simulink model "Final_v000"  (R2019b)
settings: Solver=ode4  StartTime=0.0  StopTime=10000  FixedStep=1  RelTol=1e-3
libraries: simulink x7
(part 2 of 2)

== system Final_v000/ポンプ/実H/ベルヌーイの定理/速度ヘッド ==
  v : Inport
  Constant : Constant  Value=2
  Data Store Read1 : DataStoreRead  DataStoreName=g
  Divide : Product  Inputs=*/
  Product : Product
  Square : Math  Operator=square  SignedPower=off  SaturateOnIntegerOverflow=on
  Subtract2 : Sum  Inputs=+-
  Unit Delay : UnitDelay  SampleTime=-1  HasFrameUpgradeWarning=on
  速度ヘッド : Outport
  wires:
  Constant/1 -> Product/1
  v/1 -> Square/1
  Product/1 -> Divide/2
  Unit Delay/1 -> Subtract2/2
  Square/1 -> Unit Delay/1, Subtract2/1
  Data Store Read1/1 -> Product/2
  Divide/1 -> 速度ヘッド/1
  Subtract2/1 -> Divide/1

== system Final_v000/ラジエーター/Q=hAdT/h計算/Nu更新 ==
  note: Nu=3.66 (Re<2000)
      | Nu=0.023・(Re^0.8)・(Pr^0.3) (Re>=2000)
  流量Q : Inport
  Constant : Constant  Value=3.66
  Constant1 : Constant  Value=0.023
  Constant2 : Constant  Value=0.8
  Constant3 : Constant  Value=0.3
  Power : Math  Operator=pow  SignedPower=off  SaturateOnIntegerOverflow=on
  Power1 : Math  Operator=pow  SignedPower=off  SaturateOnIntegerOverflow=on
  Product : Product  Inputs=3
  Pr更新 : Subsystem
  Re更新 : Subsystem
  Switch : Switch  Threshold=2000
  Nu : Outport
  wires:
  Constant/1 -> Switch/3
  Switch/1 -> Nu/1
  Re更新/1(Re) -> Switch/2, Power/1
  Constant2/1 -> Power/2
  Pr更新/1(Pr) -> Power1/1
  Constant3/1 -> Power1/2
  Constant1/1 -> Product/1
  Power/1 -> Product/2
  Power1/1 -> Product/3
  Product/1 -> Switch/1
  流量Q/1 -> Re更新/1(流量Q)

== system Final_v000/エンジン/Q=hAdT/h計算 /Nu更新/Pr更新 ==
  note: Pr=μ・Cp/k
  Data Store Read : DataStoreRead  DataStoreName=Cp
  Data Store Read2 : DataStoreRead  DataStoreName=viscosity
  Data Store Read3 : DataStoreRead  DataStoreName=k
  Divide : Product  Inputs=*/
  Product : Product
  Pr : Outport
  wires:
  Data Store Read2/1 -> Product/2  "μ"
  Data Store Read/1 -> Product/1  "Cp"
  Product/1 -> Divide/1
  Data Store Read3/1 -> Divide/2  "k"
  Divide/1 -> Pr/1  "Pr"

== system Final_v000/エンジン/Q=hAdT/h計算 /Nu更新/Re更新 ==
  note: Re=4ρQ/ΠμD
  流量Q : Inport
  Constant : Constant  Value=4
  Constant1 : Constant  Value=pi
  Data Store Read : DataStoreRead  DataStoreName=density
  Data Store Read2 : DataStoreRead  DataStoreName=viscosity
  Data Store Read3 : DataStoreRead  DataStoreName=D
  Divide : Product  Inputs=*/
  Product : Product  Inputs=3
  Product1 : Product  Inputs=3
  Re : Outport
  wires:
  Constant/1 -> Product/1
  Data Store Read/1 -> Product/2  "ρ"
  流量Q/1 -> Product/3  "Q"
  Product/1 -> Divide/1
  Data Store Read2/1 -> Product1/2  "μ"
  Constant1/1 -> Product1/1
  Data Store Read3/1 -> Product1/3  "D"
  Product1/1 -> Divide/2
  Divide/1 -> Re/1  "Re"

== system Final_v000/ラジエーター/Q=hAdT/h計算/Nu更新/Pr更新 ==
  note: Pr=μ・Cp/k
  Data Store Read : DataStoreRead  DataStoreName=Cp
  Data Store Read2 : DataStoreRead  DataStoreName=viscosity
  Data Store Read3 : DataStoreRead  DataStoreName=k
  Divide : Product  Inputs=*/
  Product : Product
  Pr : Outport
  wires:
  Data Store Read2/1 -> Product/2
  Data Store Read/1 -> Product/1
  Product/1 -> Divide/1
  Data Store Read3/1 -> Divide/2
  Divide/1 -> Pr/1

== system Final_v000/ラジエーター/Q=hAdT/h計算/Nu更新/Re更新 ==
  note: Re=4ρQ/ΠμD
  流量Q : Inport
  Constant : Constant  Value=4
  Constant1 : Constant  Value=pi
  Data Store Read : DataStoreRead  DataStoreName=density
  Data Store Read2 : DataStoreRead  DataStoreName=viscosity
  Data Store Read3 : DataStoreRead  DataStoreName=D
  Divide : Product  Inputs=*/
  Product : Product  Inputs=3
  Product1 : Product  Inputs=3
  Re : Outport
  wires:
  Constant/1 -> Product/1
  Data Store Read/1 -> Product/2
  流量Q/1 -> Product/3
  Product/1 -> Divide/1
  Data Store Read2/1 -> Product1/2
  Constant1/1 -> Product1/1
  Data Store Read3/1 -> Product1/3
  Product1/1 -> Divide/2
  Divide/1 -> Re/1
